simulink model "DFADAS2_SenFus_v1_201204RC_training_210115"  (R2018b)
settings: Solver=FixedStepDiscrete  StartTime=0.0  StopTime=inf  FixedStep=0.002  RelTol=1e-3  EnableMultiTasking=on
PreLoadFcn:
  | RTWConfigurationCB('preloadfcn', bdroot);
libraries: canmsglib x108, simulink x48, canfdmsglib x12
(part 23 of 28)

== system DFADAS2_SenFus_v1_201204RC_training_210115/Signal Input (Input)/Signal Input (50ms) (Input50)/Rear Left Radar(S0) Objects Information (RLRdr)/S0 Data Frame Read/Enabled Subsystem/M0ObjInfo/Subsystem1/If Action Subsystem ==
  Action Port : ActionPort  ActionType=then
  Constant : Constant  Value=0  OutDataTypeStr=uint16
  Out1 : Outport
  wires:
  Constant/1 -> Out1/1

== system DFADAS2_SenFus_v1_201204RC_training_210115/Signal Input (Input)/Signal Input (50ms) (Input50)/Rear Left Radar(S0) Objects Information (RLRdr)/S0 Data Frame Read/Enabled Subsystem/M0ObjInfo/Subsystem1/If Action Subsystem1 ==
  In1 : Inport
  Action Port : ActionPort  ActionType=else
  Out1 : Outport
  wires:
  In1/1 -> Out1/1

== system DFADAS2_SenFus_v1_201204RC_training_210115/Signal Input (Input)/Signal Input (50ms) (Input50)/Rear Left Radar(S0) Objects Information (RLRdr)/S0 Data Frame Read/Enabled Subsystem/M1ObjInfo1/Subsystem1/If Action Subsystem ==
  Action Port : ActionPort  ActionType=then
  Constant : Constant  Value=0  OutDataTypeStr=uint16
  Out1 : Outport
  wires:
  Constant/1 -> Out1/1

== system DFADAS2_SenFus_v1_201204RC_training_210115/Signal Input (Input)/Signal Input (50ms) (Input50)/Rear Left Radar(S0) Objects Information (RLRdr)/S0 Data Frame Read/Enabled Subsystem/M1ObjInfo1/Subsystem1/If Action Subsystem1 ==
  In1 : Inport
  Action Port : ActionPort  ActionType=else
  Out1 : Outport
  wires:
  In1/1 -> Out1/1

== system DFADAS2_SenFus_v1_201204RC_training_210115/Signal Input (Input)/Signal Input (50ms) (Input50)/Rear Left Radar(S0) Objects Information (RLRdr)/S0 Data Frame Read/Enabled Subsystem/M2ObjInfo/Subsystem1/If Action Subsystem ==
  Action Port : ActionPort  ActionType=then
  Constant : Constant  Value=0  OutDataTypeStr=uint16
  Out1 : Outport
  wires:
  Constant/1 -> Out1/1

== system DFADAS2_SenFus_v1_201204RC_training_210115/Signal Input (Input)/Signal Input (50ms) (Input50)/Rear Left Radar(S0) Objects Information (RLRdr)/S0 Data Frame Read/Enabled Subsystem/M2ObjInfo/Subsystem1/If Action Subsystem1 ==
  In1 : Inport
  Action Port : ActionPort  ActionType=else
  Out1 : Outport
  wires:
  In1/1 -> Out1/1

== system DFADAS2_SenFus_v1_201204RC_training_210115/Signal Input (Input)/Signal Input (50ms) (Input50)/Rear Left Radar(S0) Objects Information (RLRdr)/S0 Data Frame Read/Enabled Subsystem/M3ObjInfo/Subsystem1/If Action Subsystem ==
  Action Port : ActionPort  ActionType=then
  Constant : Constant  Value=0  OutDataTypeStr=uint16
  Out1 : Outport
  wires:
  Constant/1 -> Out1/1

== system DFADAS2_SenFus_v1_201204RC_training_210115/Signal Input (Input)/Signal Input (50ms) (Input50)/Rear Left Radar(S0) Objects Information (RLRdr)/S0 Data Frame Read/Enabled Subsystem/M3ObjInfo/Subsystem1/If Action Subsystem1 ==
  In1 : Inport
  Action Port : ActionPort  ActionType=else
  Out1 : Outport
  wires:
  In1/1 -> Out1/1

== system DFADAS2_SenFus_v1_201204RC_training_210115/Signal Input (Input)/Signal Input (50ms) (Input50)/Rear Left Radar(S0) Objects Information (RLRdr)/S0 Data Frame Read/Enabled Subsystem/M4ObjInfo1/Subsystem1/If Action Subsystem ==
  Action Port : ActionPort  ActionType=then
  Constant : Constant  Value=0  OutDataTypeStr=uint16
  Out1 : Outport
  wires:
  Constant/1 -> Out1/1

== system DFADAS2_SenFus_v1_201204RC_training_210115/Signal Input (Input)/Signal Input (50ms) (Input50)/Rear Left Radar(S0) Objects Information (RLRdr)/S0 Data Frame Read/Enabled Subsystem/M4ObjInfo1/Subsystem1/If Action Subsystem1 ==
  In1 : Inport
  Action Port : ActionPort  ActionType=else
  Out1 : Outport
  wires:
  In1/1 -> Out1/1
